simulink model "Copy_of_q4_with_control"  (R2025b)
settings: Solver=ode45  StartTime=0.0  StopTime=1200  RelTol=1e-3
settings Model: Creator=z.yin  LastModifiedBy=z.yin

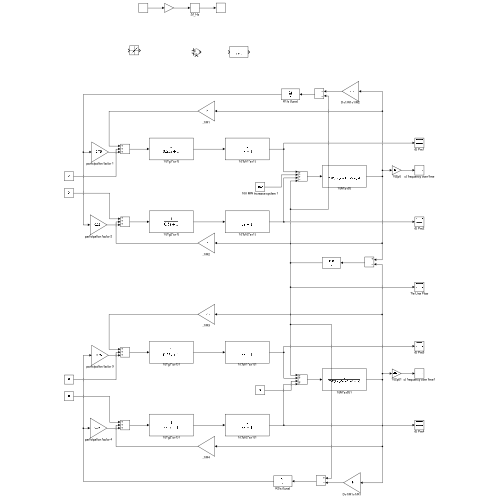
[thumbnail: Simulink's stored preview of the top-level diagram]
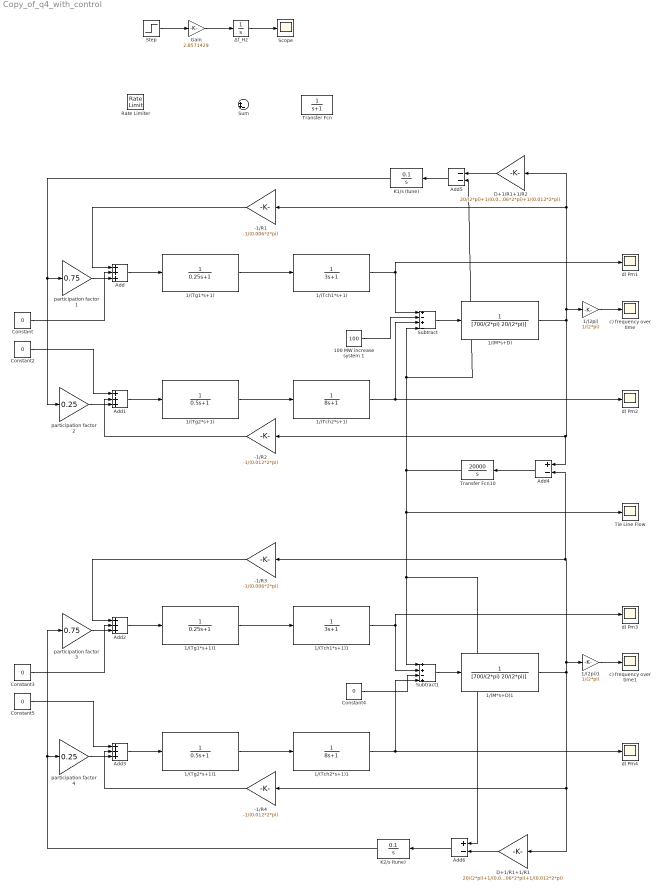
== system Copy_of_q4_with_control ==
  -1/R1 : Gain  Gain=-1/(0.006*2*pi)
  -1/R2 : Gain  Gain=-1/(0.012*2*pi)
  -1/R3 : Gain  Gain=-1/(0.006*2*pi)
  -1/R4 : Gain  Gain=-1/(0.012*2*pi)
  1/(2pi) : Gain  Gain=1/(2*pi)
  1/(2pi)1 : Gain  Gain=1/(2*pi)
  1/(M*s+D) : TransferFcn  Denominator=[700/(2*pi) 20/(2*pi)]
  1/(M*s+D)1 : TransferFcn  Denominator=[700/(2*pi) 20/(2*pi)]
  1/(Tch1*s+1) : TransferFcn  Denominator=[3 1]
  1/(Tch1*s+1)1 : TransferFcn  Denominator=[3 1]
  1/(Tch2*s+1) : TransferFcn  Denominator=[8 1]
  1/(Tch2*s+1)1 : TransferFcn  Denominator=[8 1]
  1/(Tg1*s+1) : TransferFcn  Denominator=[0.25 1]
  1/(Tg1*s+1)1 : TransferFcn  Denominator=[0.25 1]
  1/(Tg2*s+1) : TransferFcn  Denominator=[0.5 1]
  1/(Tg2*s+1)1 : TransferFcn  Denominator=[0.5 1]
  100 MW increase system 1 : Constant  Value=100
  Add{,1..3} (4 alike) : Sum  Inputs=+++
  Add4 : Sum  Inputs=+-
  Add5 : Sum  Inputs=--
  Add6 : Sum  Inputs=+-
  Constant{,2..5} (5 alike) : Constant  Value=0
  D+1/R1+1/R1 : Gain  Gain=20/(2*pi)+1/(0.006*2*pi)+1/(0.012*2*pi)
  D+1/R1+1/R2 : Gain  Gain=20/(2*pi)+1/(0.006*2*pi)+1/(0.012*2*pi)
  Gain : Gain  Gain=2.8571429
  K1/s (tune) : TransferFcn  Numerator=[0.1]  Denominator=[1 0]
  K2/s (tune) : TransferFcn  Numerator=[0.1]  Denominator=[1 0]
  Rate Limiter : RateLimiter  SampleTimeMode=inherited
  Scope : Scope
  Step : Step  Time=0  After=0.05  SampleTime=0
  Subtract : Sum  Inputs=+-+-
  Subtract1 : Sum  Inputs=++-+
  Sum : Sum  Inputs=|++-
  Tie Line Flow : Scope
      settings: ActiveDisplayYMinimum=-147.66774608789524  ActiveDisplayYMaximum=8.61997606780649  DataLoggingVariableName=Ptie
  Transfer Fcn : TransferFcn  Denominator=[1 1]
  Transfer Fcn10 : TransferFcn  Numerator=[20000]  Denominator=[1 0]
  c) frequency over time : Scope
      settings: ActiveDisplayYMinimum=-1  ActiveDisplayYMaximum=1  DataLoggingVariableName=deltaFa
  c) frequency over time1 : Scope
      settings: ActiveDisplayYMinimum=-1  ActiveDisplayYMaximum=1  DataLoggingVariableName=deltaFb
  d) Pm{1..4} (4 alike) : Scope
      d) Pm1 settings: ActiveDisplayYMinimum=-13.79191550661649  ActiveDisplayYMaximum=97.653496118051692  DataLoggingVariableName=Pm1
      d) Pm2 settings: ActiveDisplayYMinimum=-3.9741691062345192  ActiveDisplayYMaximum=35.767521956110684  DataLoggingVariableName=Pm2
      d) Pm3 settings: ActiveDisplayYMinimum=-13.79191550661649  ActiveDisplayYMaximum=97.653496118051692  DataLoggingVariableName=Pm3
      d) Pm4 settings: ActiveDisplayYMinimum=-3.9741691062345192  ActiveDisplayYMaximum=35.767521956110684  DataLoggingVariableName=Pm4
  participation factor 1 : Gain  Gain=0.75
  participation factor 2 : Gain  Gain=0.25
  participation factor 3 : Gain  Gain=0.75
  participation factor 4 : Gain  Gain=0.25
  Δf_Hz : Integrator
  wires:
  Step/1 -> Gain/1
  Gain/1 -> Δf_Hz/1
  Δf_Hz/1 -> Scope/1
  1/(Tg2*s+1)/1 -> 1/(Tch2*s+1)/1
  1/(Tch2*s+1)/1 -> d) Pm2/1, Subtract/3
  1/(Tg1*s+1)/1 -> 1/(Tch1*s+1)/1
  100 MW increase system 1/1 -> Subtract/2
  Add1/1 -> 1/(Tg2*s+1)/1
  1/(Tch1*s+1)/1 -> d) Pm1/1, Subtract/1
  Constant2/1 -> Add1/1
  -1/R2/1 -> Add1/2
  1/(2pi)/1 -> c) frequency over time/1
  Subtract/1 -> 1/(M*s+D)/1
  -1/R1/1 -> Add/1
  Add/1 -> 1/(Tg1*s+1)/1
  Constant/1 -> Add/2
  K1/s (tune)/1 -> participation factor 2/1, participation factor 1/1
  participation factor 2/1 -> Add1/3
  participation factor 1/1 -> Add/3
  -1/R4/1 -> Add3/2
  1/(Tch2*s+1)1/1 -> Subtract1/4, d) Pm4/1
  Add3/1 -> 1/(Tg2*s+1)1/1
  1/(Tg1*s+1)1/1 -> 1/(Tch1*s+1)1/1
  Subtract1/1 -> 1/(M*s+D)1/1
  Constant4/1 -> Subtract1/3
  1/(Tg2*s+1)1/1 -> 1/(Tch2*s+1)1/1
  Constant3/1 -> Add2/2
  Constant5/1 -> Add3/1
  Add2/1 -> 1/(Tg1*s+1)1/1
  participation factor 4/1 -> Add3/3
  1/(2pi)1/1 -> c) frequency over time1/1
  -1/R3/1 -> Add2/1
  K2/s (tune)/1 -> participation factor 3/1, participation factor 4/1
  participation factor 3/1 -> Add2/3
  1/(Tch1*s+1)1/1 -> Subtract1/2, d) Pm3/1
  1/(M*s+D)/1 -> Add4/1, -1/R2/1, 1/(2pi)/1, -1/R1/1, D+1/R1+1/R2/1
  1/(M*s+D)1/1 -> D+1/R1+1/R1/1, -1/R4/1, Add4/2, -1/R3/1, 1/(2pi)1/1
  Add4/1 -> Transfer Fcn10/1
  Transfer Fcn10/1 -> Add6/1, Subtract1/1, Tie Line Flow/1, Subtract/4, Add5/2
  D+1/R1+1/R2/1 -> Add5/1
  Add5/1 -> K1/s (tune)/1
  D+1/R1+1/R1/1 -> Add6/2
  Add6/1 -> K2/s (tune)/1
